simulink model "bank_system"  (R2020a)
settings: Solver=VariableStepAuto  StartTime=0.0  StopTime=10.0  RelTol=1e-3
values from neighbouring files (symbols this model uses):
  i_l = 0.075    [bank_and_economy.m]    (also in bank_centralbank.m = 0.055; bootstrapping.m = 0.055; main.m = 0.055)
  i_m = 0.03    [bank_and_economy.m]    (also in bank_centralbank.m; bootstrapping.m; main.m)
  K_0 = 0.08    [a_1.m]    (also in a_2.m; a_loss_function.m; bank_and_economy.m; bank_centralbank.m)
  K_p = 15    [a_1.m]    (also in a_2.m; a_loss_function.m; bank_and_economy.m = 0.5; bank_centralbank.m)
  lambda = 0.002    [a_1.m]    (also in a_2.m; a_loss_function.m; bank_and_economy.m; bank_centralbank.m)
  R = 1    [a_1.m]    (also in a_2.m; a_loss_function.m; bank_and_economy.m; bank_centralbank.m)
  rate = 0.1    [a_1.m]    (also in a_2.m; a_loss_function.m; bank_and_economy.m; bank_centralbank.m)
  sigma = 0.28    [a_1.m]    (also in a_2.m; a_loss_function.m; bank_and_economy.m; bank_centralbank.m)
  T_i = 8    [a_1.m]    (also in a_2.m; a_loss_function.m; bank_and_economy.m; bank_centralbank.m)
libraries: simulink x1
settings Model: Creator=erlended  LastModifiedBy=erlended

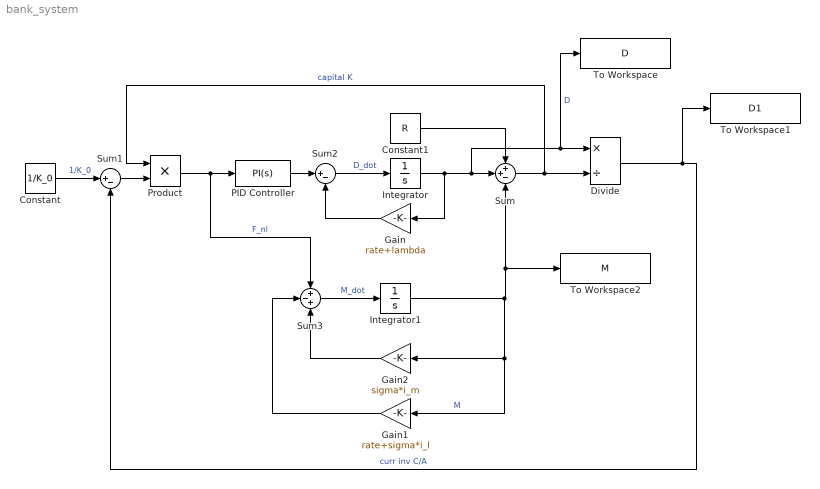
== system bank_system ==
  Constant : Constant  Value=1/K_0
  Constant1 : Constant  Value=R
  Divide : Product  Inputs=*/
  Gain : Gain  Gain=rate+lambda
  Gain1 : Gain  Gain=rate+sigma*i_l
  Gain2 : Gain  Gain=sigma*i_m
  Integrator : Integrator
  Integrator1 : Integrator
  PID Controller : simulink/Continuous/PID Controller  Controller=PI  Form=Parallel  TimeDomain=Continuous-time  UseExternalTs=off  SampleTime=-1  IntegratorMethod=Forward Euler  FilterMethod=Forward Euler  ControllerParametersSource=internal  P=K_p  I=(1+T_i)/T_i  D=0  UseFilter=on  N=100  TunerSelectOption=Transfer Function Based (PID Tuner App)  InitialConditionSource=internal  InitialConditionForIntegrator=0  InitialConditionForFilter=0  DifferentiatorICPrevScaledInput=0  ExternalReset=none  TrackingMode=off  Kt=1  LimitOutput=off  UpperSaturationLimit=inf  LowerSaturationLimit=-inf  LinearizeAsGain=on  AntiWindupMode=none  Kb=1  POutMin=[]  POutMax=[]  IOutMin=[]  IOutMax=[]  DOutMin=[]  DOutMax=[]  NOutMin=[]  NOutMax=[]  SumOutMin=[]  SumOutMax=[]  SaturationOutMin=[]  SaturationOutMax=[]  PParamMin=[]  PParamMax=[]  IParamMin=[]  IParamMax=[]  DParamMin=[]  DParamMax=[]  NParamMin=[]  NParamMax=[]  KbParamMin=[]  KbParamMax=[]  KtParamMin=[]  KtParamMax=[]  KbOutMin=[]  KbOutMax=[]  KtOutMin=[]  KtOutMax=[]  IntegratorOutMin=[]  IntegratorOutMax=[]  FilterOutMin=[]  FilterOutMax=[]  SumI1OutMin=[]  SumI1OutMax=[]  SumI2OutMin=[]  SumI2OutMax=[]  SumI3OutMin=[]  SumI3OutMax=[]  SumI4OutMin=[]  SumI4OutMax=[]  SumDOutMin=[]  SumDOutMax=[]  DifferentiatorOutMin=[]  DifferentiatorOutMax=[]  FilterDiffOutCoefMin=[]  FilterDiffOutCoefMax=[]  ReciprocalOutMin=[]  ReciprocalOutMax=[]  SumDenOutMin=[]  SumDenOutMax=[]  SumNumOutMin=[]  SumNumOutMax=[]  DivideOutMin=[]  DivideOutMax=[]  UdiffTsProdOutMin=[]  UdiffTsProdOutMax=[]  NTsProdOutMin=[]  NTsProdOutMax=[]  UintegralTsProdOutMin=[]  UintegralTsProdOutMax=[]  UngainTsProdOutMin=[]  UngainTsProdOutMax=[]  IntegratorContinuousStateAttributes=''  IntegratorStateMustResolveToSignalObject=off  IntegratorRTWStateStorageClass=Auto  FilterContinuousStateAttributes=''  FilterStateMustResolveToSignalObject=off  FilterRTWStateStorageClass=Auto  ParallelPVariant=InternalParameters  IdealPVariant=Disabled  IVariant=InternalParameters  DVariant=Disabled  IntegratorVariant=Continuous  SatVariant=Disabled  AWVariant=Passthrough  PCopyVariant=Disabled  TRVariant=Disabled  FdbkBlocksVariant=Forward  IdealPFdbkVariant=Disabled  SatFdbkVariant=Disabled  DerivativeFilterVariant=Disabled  NVariant=Disabled  NCopyVariant=Disabled_SignalSpec  FilterICVariant=Disabled  IntegratorICVariant=InternalICs  ExternalResetVariant=Disabled  TRSumVariant=Passthrough  SumFdbkVariant=Disabled  SumVariant=Sum_PI  TsampFilterVariant=InternalTs  TsampNgainVariant=Passthrough  TsampIntegralVariant=Passthrough
  Product : Product
  Sum : Sum  Inputs=++-
  Sum1 : Sum  Inputs=|+-
  Sum2 : Sum  Inputs=|+-
  Sum3 : Sum  Inputs=+-+
  To Workspace : ToWorkspace  VariableName=D  SaveFormat=Timeseries  SampleTime=-1
  To Workspace1 : ToWorkspace  VariableName=D1  SaveFormat=Timeseries  SampleTime=-1
  To Workspace2 : ToWorkspace  VariableName=M  SaveFormat=Timeseries  SampleTime=-1
  wires:
  Product/1 -> Sum3/1, PID Controller/1  "F_nl"
  Sum/1 -> Product/1, Divide/2  "capital K"
  Sum1/1 -> Product/2
  Constant/1 -> Sum1/1  "1/K_0"
  PID Controller/1 -> Sum2/1
  Sum2/1 -> Integrator/1  "D_dot"
  Integrator/1 -> Gain/1, To Workspace/1, Divide/1, Sum/2  "D"
  Constant1/1 -> Sum/1
  Gain/1 -> Sum2/2
  Integrator1/1 -> Gain2/1, Gain1/1, To Workspace2/1, Sum/3  "M"
  Sum3/1 -> Integrator1/1  "M_dot"
  Gain1/1 -> Sum3/2
  Gain2/1 -> Sum3/3
  Divide/1 -> To Workspace1/1, Sum1/2  "curr inv C/A"
